simulink model "MotorDC"  (R2021a)
settings: Solver=VariableStepAuto  StartTime=0.0  StopTime=1  RelTol=1e-3
values from neighbouring files (symbols this model uses):
  B = [0; 0; w^2*b; 0]    [Avion.m]    (also in MotorCC.m = 0; RLC.m = [1/L ;0])
  J = 5e-9    (= 5e-09)    [MotorCC.m]
  Ki = 0.833    [MotorCC.m]
  Km = 60e-3    (= 0.06)    [MotorCC.m]
  Laa = 366e-6    (= 0.000366)    [MotorCC.m]
  Ra = 100    [MotorCC.m]
settings Model: Creator=bruno  LastModifiedBy=bruno

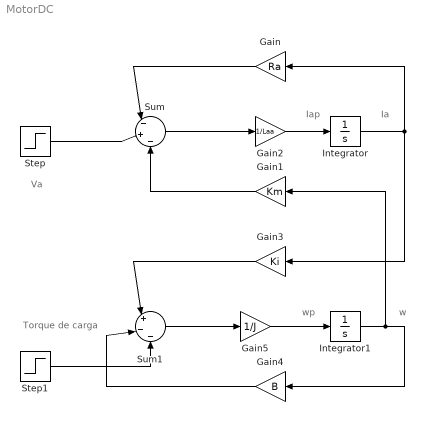
== system MotorDC ==
  note: Iap
  note: wp
  note: w
  note: Ia
  note: Torque de carga
  note: Va
  Gain : Gain  Gain=Ra
  Gain1 : Gain  Gain=Km
  Gain2 : Gain  Gain=1/Laa
  Gain3 : Gain  Gain=Ki
  Gain4 : Gain  Gain=B
  Gain5 : Gain  Gain=1/J
  Integrator : Integrator
  Integrator1 : Integrator
  Step : Step  Time=0  After=12  SampleTime=0
  Step1 : Step  Time=0.1  After=0.075  SampleTime=0
  Sum : Sum  Inputs=|-|+|-
  Sum1 : Sum  Inputs=|+|-|-
  wires:
  Gain/1 -> Sum/1
  Step/1 -> Sum/2
  Gain1/1 -> Sum/3
  Sum/1 -> Gain2/1
  Gain2/1 -> Integrator/1
  Integrator/1 -> Gain3/1, Gain/1
  Sum1/1 -> Gain5/1
  Gain4/1 -> Sum1/2
  Integrator1/1 -> Gain1/1, Gain4/1
  Gain3/1 -> Sum1/1
  Gain5/1 -> Integrator1/1
  Step1/1 -> Sum1/3
